simulink model "finalsimulink"  (R2026a)
settings: Solver=ode45  StopTime=20  MaxStep=0.0001
values from neighbouring files (symbols this model uses):
  LUT_Cd = [t_cd,  Cd_val]    [init_lookup_tables.m]
  LUT_Cm = [t_cm,  Cm_val]    [init_lookup_tables.m]
  LUT_Cp = [t_cp,  Cp_val]    [init_lookup_tables.m]
  LUT_Fn = [t_fn,  Fn_val]    [init_lookup_tables.m]
  LUT_Thrust = [t_thr, T_val]    [init_lookup_tables.m]
  m_water_prop = 0.5    [rocket_params.m]
libraries: slident x1
settings Model: Creator=marti  LastModifiedBy=marti

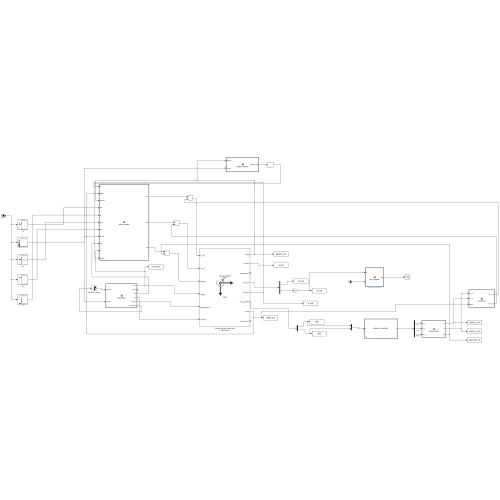
[thumbnail: Simulink's stored preview of the top-level diagram]
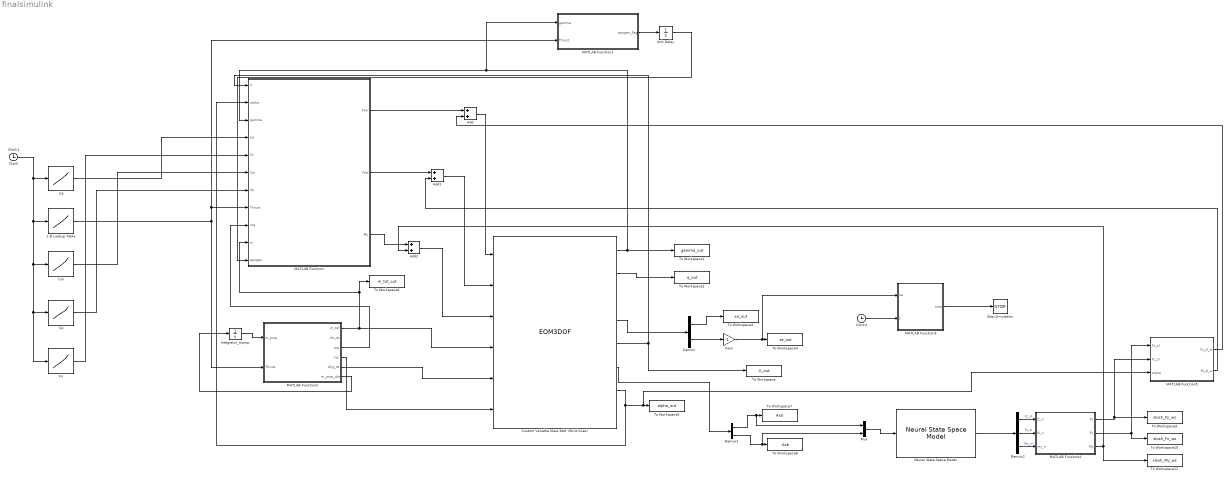
== system finalsimulink ==
  1-D Lookup Table : Lookup_n-D  NumberOfTableDimensions=1  BreakpointsForDimension1=LUT_Thrust(:,1)  Table=LUT_Thrust(:,2)  ExtrapMethod=Clip  InternalRulePriority=Speed  RndMeth=Simplest
  Add : Sum
  Add1 : Sum
  Add2 : Sum
  Cd : Lookup_n-D  NumberOfTableDimensions=1  BreakpointsForDimension1=LUT_Cd(:,1)  Table=LUT_Cd(:,2)  ExtrapMethod=Clip  InternalRulePriority=Speed  RndMeth=Simplest
  Clock : Clock
  Clock1 : Clock
  Clock2 : Clock
  Cm : Lookup_n-D  NumberOfTableDimensions=1  BreakpointsForDimension1=LUT_Cm(:,1)  Table=LUT_Cm(:,2)  ExtrapMethod=Clip  InternalRulePriority=Speed  RndMeth=Simplest
  Cp : Lookup_n-D  NumberOfTableDimensions=1  BreakpointsForDimension1=LUT_Cp(:,1)  Table=LUT_Cp(:,2)  ExtrapMethod=Clip  InternalRulePriority=Speed  RndMeth=Simplest
  Custom Variable Mass 3dof (Wind Axes) : EOM3DOF  axes=Wind  mtype=Custom Variable  v_ini=0.001  gamma_ini=(88*pi)/180  abi_flag=on
  Demux : Demux  Outputs=2
  Demux1 : Demux  Outputs=2
  Demux2 : Demux  Outputs=3
  Fn : Lookup_n-D  NumberOfTableDimensions=1  BreakpointsForDimension1=LUT_Fn(:,1)  Table=LUT_Fn(:,2)  ExtrapMethod=Clip  InternalRulePriority=Speed  RndMeth=Simplest
  Gain : Gain  Gain=-1
  Integrator_mprop : Integrator  InitialCondition=m_water_prop  LimitOutput=on  LowerSaturationLimit=0
  MATLAB Function : MATLAB Function  TreatAsAtomicUnit=on
  MATLAB Function1 : MATLAB Function  TreatAsAtomicUnit=on
  MATLAB Function2 : MATLAB Function  TreatAsAtomicUnit=on
  MATLAB Function3 : MATLAB Function  TreatAsAtomicUnit=on
  MATLAB Function4 : MATLAB Function  TreatAsAtomicUnit=on
  MATLAB Function5 : MATLAB Function  TreatAsAtomicUnit=on
  Mux : Mux  Inputs=2
  Neural State Space Model : slident/Models/Neural State Space Model  sys=sys_nss_trained  x0type=internal  ic=[0 0]  returnx=off  returndx=off
  Stop Simulation : Stop
  To Workspace : ToWorkspace  VariableName=V_out  SampleTime=-1
  To Workspace1 : ToWorkspace  VariableName=gamma_out  SampleTime=-1
  To Workspace10 : ToWorkspace  VariableName=slosh_Fx_ws  SampleTime=-1
  To Workspace11 : ToWorkspace  VariableName=slosh_My_ws  SampleTime=-1
  To Workspace2 : ToWorkspace  VariableName=q_out  SampleTime=-1
  To Workspace3 : ToWorkspace  VariableName=xe_out  SampleTime=-1
  To Workspace4 : ToWorkspace  VariableName=ze_out  SampleTime=-1
  To Workspace5 : ToWorkspace  VariableName=alpha_out  SampleTime=-1
  To Workspace6 : ToWorkspace  VariableName=m_tot_out  SampleTime=-1
  To Workspace7 : ToWorkspace  VariableName=Axb  SampleTime=-1
  To Workspace8 : ToWorkspace  VariableName=Azb  SampleTime=-1
  To Workspace9 : ToWorkspace  VariableName=slosh_Fz_ws  SampleTime=-1
  Unit Delay : UnitDelay  SampleTime=-1
  wires:
  Clock1/1 -> 1-D Lookup Table/1, Fn/1, Cp/1, Cm/1, Cd/1
  Integrator_mprop/1 -> MATLAB Function2/1(m_prop)
  1-D Lookup Table/1 -> MATLAB Function2/2(Thrust), MATLAB Function/8(Thrust), MATLAB Function1/2(Thrust)
  MATLAB Function2/1(m_tot) -> Custom Variable Mass 3dof (Wind Axes)/4, To Workspace6/1, MATLAB Function/10(m)
  Custom Variable Mass 3dof (Wind Axes)/4 -> Demux/1
  Custom Variable Mass 3dof (Wind Axes)/1 -> MATLAB Function1/1(gamma), MATLAB Function/3(gamma), To Workspace1/1
  Custom Variable Mass 3dof (Wind Axes)/2 -> To Workspace2/1
  Demux/1 -> To Workspace3/1
  Demux/2 -> Gain/1
  Custom Variable Mass 3dof (Wind Axes)/7 -> MATLAB Function/2(alpha), MATLAB Function5/3(alpha), To Workspace5/1
  Cd/1 -> MATLAB Function/4(Cd)
  Fn/1 -> MATLAB Function/5(Fn)
  Cm/1 -> MATLAB Function/6(Cm)
  Cp/1 -> MATLAB Function/7(Cp)
  MATLAB Function2/3(xcg) -> MATLAB Function/9(xcg)
  Custom Variable Mass 3dof (Wind Axes)/5 -> To Workspace/1, MATLAB Function/1(V)
  MATLAB Function1/1(apogeo_flag) -> Unit Delay/1
  Unit Delay/1 -> MATLAB Function/11(apogeo)
  Gain/1 -> MATLAB Function3/1(ze), To Workspace4/1
  MATLAB Function2/6(m_prop_dot) -> Integrator_mprop/1
  MATLAB Function2/4(Iyy) -> Custom Variable Mass 3dof (Wind Axes)/6
  MATLAB Function2/5(dIyy_dt) -> Custom Variable Mass 3dof (Wind Axes)/5
  MATLAB Function3/1(stop) -> Stop Simulation/1
  Clock2/1 -> MATLAB Function3/2(t)
  Custom Variable Mass 3dof (Wind Axes)/6 -> Demux1/1
  Demux1/1 -> Mux/1, To Workspace7/1
  Demux1/2 -> Mux/2, To Workspace8/1
  Mux/1 -> Neural State Space Model/1
  Neural State Space Model/1 -> Demux2/1
  Demux2/1 -> MATLAB Function4/1(fz_n)  "Fz_sl"
  Demux2/2 -> MATLAB Function4/2(fx_n)  "Fx_sl"
  Demux2/3 -> MATLAB Function4/3(my_n)  "My_sl"
  MATLAB Function4/1(Fz) -> To Workspace9/1, MATLAB Function5/2(Fz_sl)
  MATLAB Function4/2(Fx) -> To Workspace10/1, MATLAB Function5/1(Fx_sl)
  MATLAB Function/1(Fxw) -> Add/1
  MATLAB Function5/1(Fx_sl_w) -> Add/2
  Add/1 -> Custom Variable Mass 3dof (Wind Axes)/1
  MATLAB Function/2(Fzw) -> Add1/1
  MATLAB Function5/2(Fz_sl_w) -> Add1/2
  Add1/1 -> Custom Variable Mass 3dof (Wind Axes)/2
  MATLAB Function4/3(My) -> To Workspace11/1, Add2/2
  MATLAB Function/3(My) -> Add2/1
  Add2/1 -> Custom Variable Mass 3dof (Wind Axes)/3

== matlab function finalsimulink/MATLAB Function ==
  data: V input; Fxw output; alpha input; gamma input; Cd input; Fn input; Cm input; Cp input; Thrust input; xcg input; m input; Fzw output; My output; apogeo input
function [Fxw, Fzw, My] = forze_momenti(V, alpha, gamma, Cd, Fn, Cm, Cp, Thrust, xcg, m, apogeo)
    
    % 1. PRE-ALLOCAZIONE RIGIDA
    Fxw = 0.0;
    Fzw = 0.0;
    My  = 0.0;

    %% Parametri fissi
    rho      = 1.225;
    g0       = 9.81;
    A_ref    = pi * 0.055^2;
    D_ref    = 0.11;
    Cd_chute = 0.8;
    A_chute  = pi * 0.5^2;

    %% Velocità scalare con protezione
    V_scalar = V(1); 
    V_eff    = max(V_scalar, 0.5); 
    q_dyn    = 0.5 * rho * V_eff^2;

    %% Forze Aerodinamiche (Asse Vento)
    FA = q_dyn * A_ref * Cd;      
    FL = q_dyn * A_ref * Fn;      

    %% Spinta
    Fx_thrust =  Thrust * cos(alpha);
    Fz_thrust = -Thrust * sin(alpha); 

    %% Paracadute
    F_chute = apogeo * (0.5 * rho * V_scalar^2 * Cd_chute * A_chute);

    %% Equazioni totali in Assi Vento
    Fxw = Fx_thrust - FA - F_chute;
    Fzw = -FL + Fz_thrust;

    %% Momento di Beccheggio
    arm = xcg - Cp;
    
    if apogeo == 0
        My = q_dyn * A_ref * D_ref * Cm + FL * arm;
    else
        My = 0; 
    end
end

== matlab function finalsimulink/MATLAB Function2 ==
  data: m_prop input; m_tot output; Thrust input; dm_dt output; xcg output; Iyy output; dIyy_dt output; m_prop_dot output
function [m_tot, dm_dt, xcg, Iyy, dIyy_dt, m_prop_dot] = MassAndCG(m_prop, Thrust)

%% Dichiarazioni dimensioni output — obbligatorio per Simulink
m_tot      = 0.0;
dm_dt      = 0.0;
xcg        = 0.0;
Iyy        = 0.0;
dIyy_dt    = 0.0;
m_prop_dot = 0.0;

    %% Parametri fissi
    g0            = 9.81;
    Isp_eff       = 7.5;
    m_dry         = 0.945;
    m_water_pay   = 0.5;
    L_rocket      = 1.00;
    R_rocket      = 0.055;
    xcg_dry       = 0.50;
    xcg_tank_prop = 0.85;
    xcg_tank_pay  = 0.35;
    L_tank        = 0.30;

    %% Massa propellente con protezione numerica
    m_prop_safe = max(m_prop, 0);

    %% Massa totale
    m_tot = m_dry + m_prop_safe + m_water_pay;

    %% Rateo di variazione massa
    if m_prop_safe > 1e-6 && Thrust > 1.0
        m_prop_dot = -Thrust / (Isp_eff * g0);
    else
        m_prop_dot = 0.0;
    end
    dm_dt = m_prop_dot;

    %% Posizione CG composta
    xcg = (m_dry * xcg_dry + m_prop_safe * xcg_tank_prop + ...
           m_water_pay * xcg_tank_pay) / m_tot;

    %% Momento d'inerzia scalare
    Iyy_dry    = m_dry        * (3*R_rocket^2 + L_rocket^2) / 12;
    Iyy_prop   = m_prop_safe  * (3*R_rocket^2 + L_tank^2)   / 12;
    Iyy_pay    = m_water_pay  * (3*R_rocket^2 + L_tank^2)   / 12;

    Iyy_scalar = Iyy_dry  + m_dry        * (xcg - xcg_dry)^2       + ...
                 Iyy_prop + m_prop_safe   * (xcg - xcg_tank_prop)^2 + ...
                 Iyy_pay  + m_water_pay   * (xcg - xcg_tank_pay)^2;

    dIyy_scalar = m_prop_dot * (3*R_rocket^2 + L_tank^2) / 12 + ...
                  m_prop_dot * (xcg - xcg_tank_prop)^2;

    %% Output scalari — verranno uniti da Mux nel canvas
    %% Output — tutti scalari
Iyy     = Iyy_scalar;
dIyy_dt = dIyy_scalar;

end

== matlab function finalsimulink/MATLAB Function1 ==
  settings: updateMethod=DISCRETE  sampleTime=0.001
  data: gamma input; apogeo_flag output; Thrust input
function apogeo_flag = apogeo_detector(gamma, Thrust)
    % persistent mantiene lo stato tra un passo di simulazione e l'altro
    persistent flag counter
    
    if isempty(flag)
        flag = 0;
        counter = 0; % Contatore per la conferma software dell'apogeo
    end
    
    % Se l'apogeo è già stato rilevato, blocca il flag a 1 e bypassa i calcoli
    if flag == 1
        apogeo_flag = 1;
        return;
    end
    
    %% Condizione di Apogeo con filtro anti-rumore
    % 1. La spinta deve essere terminata (Thrust < 0.1 N)
    % 2. L'angolo di traiettoria deve essere significativamente negativo (es. < -1 grado)
    %    Convertiamo -1° in radianti: -1 * pi / 180 = -0.0175 rad
    
    if Thrust < 0.1 && gamma < -0.0175
        counter = counter + 1;
    else
        counter = max(0, counter - 1); % Se è stato un falso allarme, resetta lentamente
    end
    
    % Se la condizione persiste per almeno 5 passi consecutivi del solver,
    % allora l'apogeo è reale e confermato.
    if counter >= 5
        flag = 1;
    end
    
    apogeo_flag = flag;
end

== matlab function finalsimulink/MATLAB Function3 ==
  data: ze input; stop output; t input
function stop = stop_condition(ze, t)
    % Stoppa quando il razzo torna a quota 0 dopo il lancio
    if t > 2.0 && ze <= 0
        stop = 1.0;
    else
        stop = 0.0;
    end
end

== matlab function finalsimulink/MATLAB Function4 ==
  data: fz_n input; Fz output; Fx output; fx_n input; my_n input; My output
 function [Fz, Fx, My] = denormalizza(fz_n, fx_n, my_n)
        mu_out  = [-0.000346,  0.004512, -0.000191];
        std_out = [ 0.152827,  0.010912,  0.044635];

        Fz = fz_n * std_out(1) + mu_out(1);
        Fx = fx_n * std_out(2) + mu_out(2);
        My = my_n * std_out(3) + mu_out(3);

        % Saturazione ai valori massimi fisici del training
        Fz = max(min(Fz,  2.47), -2.47);
        Fx = max(min(Fx,  6.75), -6.75);
        My = max(min(My,  2.03), -2.03);
    end

== matlab function finalsimulink/MATLAB Function5 ==
  data: Fx_sl input; Fx_sl_w output; Fz_sl input; alpha input; Fz_sl_w output
function [Fx_sl_w, Fz_sl_w] = body2wind(Fx_sl, Fz_sl, alpha)
        Fx_sl_w =  Fx_sl * cos(alpha) + Fz_sl * sin(alpha);
        Fz_sl_w = -Fx_sl * sin(alpha) + Fz_sl * cos(alpha);
end
